simulink model "lab12_KE_Analysis"  (R2025a)
settings: Solver=VariableStepAuto  StartTime=0.0  StopTime=10  RelTol=1e-3
settings Model: Creator=hp  LastModifiedBy=hp

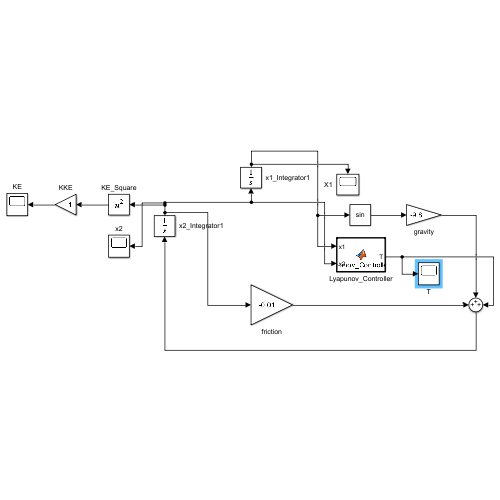
[thumbnail: Simulink's stored preview of the top-level diagram]
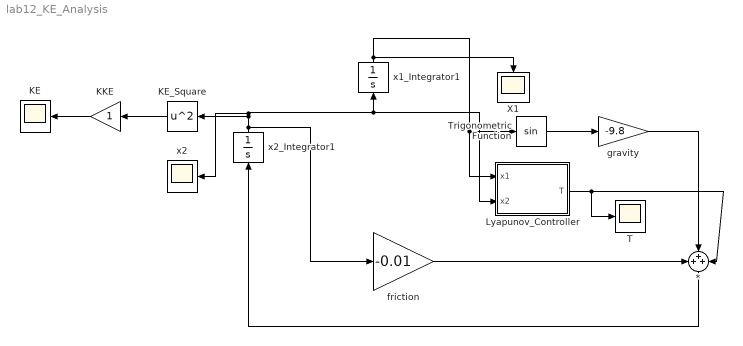
== system lab12_KE_Analysis ==
  * : Sum  Inputs=+++
  KE : Scope
      settings: ActiveDisplayYMinimum=-0.12499999999999997  ActiveDisplayYMaximum=1.125  DataLoggingVariableName=ScopeData3
  KE_Square : Math  Operator=square
  KKE : Gain
  Lyapunov_Controller : MATLAB Function  TreatAsAtomicUnit=on
  T : Scope
      settings: ActiveDisplayYMinimum=5.8165362495191717  ActiveDisplayYMaximum=10.215330265501322  DataLoggingVariableName=ScopeData2
  Trigonometric Function : Trigonometry
  X1 : Scope
      settings: ActiveDisplayYMinimum=-1.8357182296887213  ActiveDisplayYMaximum=1.9874438481497838
  friction : Gain  Gain=-0.01
  gravity : Gain  Gain=-9.8
  x1_Integrator1 : Integrator  InitialCondition=1
  x2 : Scope
      settings: ActiveDisplayYMinimum=-0.12499999768095674  ActiveDisplayYMaximum=1.1249999997423286
  x2_Integrator1 : Integrator  InitialCondition=1
  wires:
  KKE/1 -> KE/1
  KE_Square/1 -> KKE/1
  x2_Integrator1/1 -> x1_Integrator1/1, Lyapunov_Controller/2(x2), x2/1, KE_Square/1, friction/1
  x1_Integrator1/1 -> Lyapunov_Controller/1(x1), Trigonometric Function/1, X1/1
  Lyapunov_Controller/1(T) -> */3, T/1
  friction/1 -> */1
  gravity/1 -> */2
  Trigonometric Function/1 -> gravity/1
  */1 -> x2_Integrator1/1

== matlab function lab12_KE_Analysis/Lyapunov_Controller ==
  data: T output; x1 input; x2 input
function T = Lyapunov_Controller_B(x1, x2)

Kd = 2;

T = 9.8*sin(x1) + 0.01*x2 - Kd*x2;

end
